simulink model "Integration_1_1"  (R2024b)
settings: Solver=VariableStepAuto  StartTime=0.0  StopTime=4  RelTol=1e-3
undefined symbols (not defined in the file): Ion, Lithium, Ts_Control
libraries: ee_lib x30, nesl_utility x24, spsSeriesRLCBranchLib x22, simulink x21, slpidlib x18, spsParallelRLCBranchLib x18, spsCurrentVoltageSimscapeInterfaceLib x18, powerlib_extras x18, spsThreePhaseVIMeasurementLib x7, spsGroundLib x7, spsThreePhaseSeriesRLCBranchLib x7, spsBoostConverterLib x6
(part 1 of 5)
settings Model: Creator=DELL  LastModifiedBy=mitphanase
settings DataIOCC: ReturnWorkspaceOutputs=off

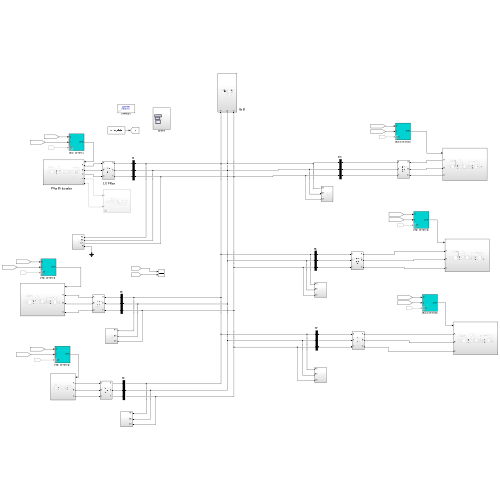
[thumbnail: Simulink's stored preview of the top-level diagram]
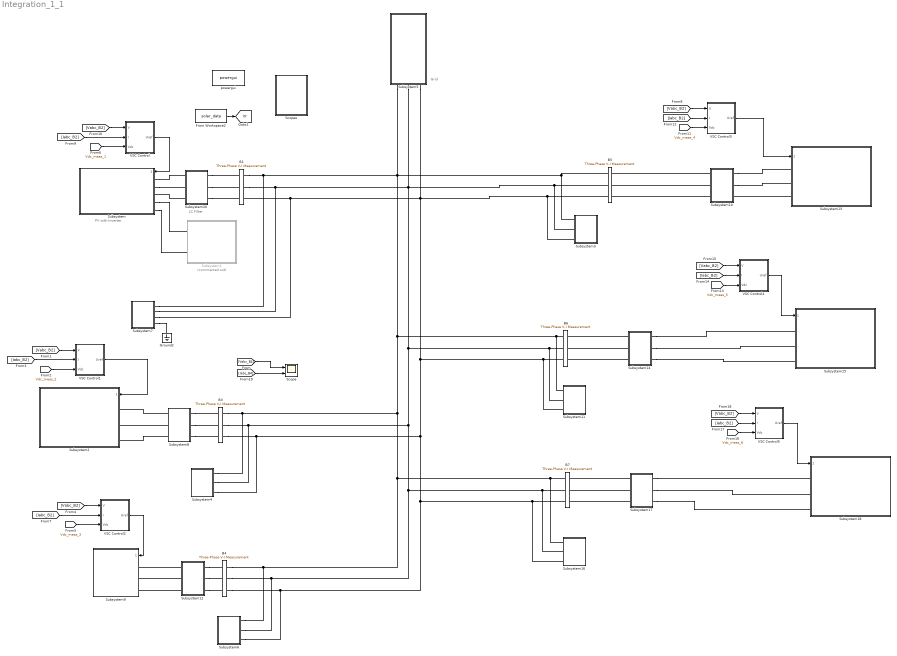
== system Integration_1_1 ==
  note: LC Filter
  note: Grid
  note: PV with Inverter
  B1 : spsThreePhaseVIMeasurementLib/Three-Phase V-I Measurement  VoltageMeasurement=phase-to-ground  SetLabelV=on  LabelV=Vabc_B1  Vpu=off  VpuLL=off  CurrentMeasurement=yes  SetLabelI=on  LabelI=Iabc_B1  Ipu=off  Pbase=100e6  Vbase=1000  OutputType=Magnitude  PhasorSimulation=off  PSBequivalent=0
  B3 : spsThreePhaseVIMeasurementLib/Three-Phase V-I Measurement  VoltageMeasurement=phase-to-ground  SetLabelV=on  LabelV=Vabc_B3  Vpu=off  VpuLL=off  CurrentMeasurement=yes  SetLabelI=on  LabelI=Iabc_B3  Ipu=off  Pbase=100e6  Vbase=1000  OutputType=Magnitude  PhasorSimulation=off  PSBequivalent=0
  B4 : spsThreePhaseVIMeasurementLib/Three-Phase V-I Measurement  VoltageMeasurement=phase-to-phase  SetLabelV=on  LabelV=Vabc_B4  Vpu=off  VpuLL=off  CurrentMeasurement=yes  SetLabelI=on  LabelI=Iabc_B4  Ipu=off  Pbase=100e6  Vbase=1000  OutputType=Magnitude  PhasorSimulation=off  PSBequivalent=0
  B5 : spsThreePhaseVIMeasurementLib/Three-Phase V-I Measurement  VoltageMeasurement=phase-to-phase  SetLabelV=on  LabelV=Vabc_B5  Vpu=off  VpuLL=off  CurrentMeasurement=yes  SetLabelI=on  LabelI=Iabc_B5  Ipu=off  Pbase=100e6  Vbase=1000  OutputType=Magnitude  PhasorSimulation=off  PSBequivalent=0
  B6 : spsThreePhaseVIMeasurementLib/Three-Phase V-I Measurement  VoltageMeasurement=phase-to-phase  SetLabelV=on  LabelV=Vabc_B6  Vpu=off  VpuLL=off  CurrentMeasurement=yes  SetLabelI=on  LabelI=Iabc_B6  Ipu=off  Pbase=100e6  Vbase=1000  OutputType=Magnitude  PhasorSimulation=off  PSBequivalent=0
  B7 : spsThreePhaseVIMeasurementLib/Three-Phase V-I Measurement  VoltageMeasurement=phase-to-phase  SetLabelV=on  LabelV=Vabc_B7  Vpu=off  VpuLL=off  CurrentMeasurement=yes  SetLabelI=on  LabelI=Iabc_B7  Ipu=off  Pbase=100e6  Vbase=1000  OutputType=Magnitude  PhasorSimulation=off  PSBequivalent=0
  From Workspace2 : FromWorkspace  VariableName=solar_data  OutDataTypeStr=double  SampleTime=0.01
  Ground2 : spsGroundLib/Ground  LConnTagsString=a
  Scope : Scope  NumInputPorts=2
  Scopes : Subsystem
  Subsystem : Subsystem
  Subsystem1 : Subsystem  Commented=on
  Subsystem10 : Subsystem
  Subsystem11 : Subsystem
  Subsystem12 : Subsystem
  Subsystem13 : Subsystem
  Subsystem14 : Subsystem
  Subsystem15 : Subsystem
  Subsystem16 : Subsystem
  Subsystem17 : Subsystem
  Subsystem18 : Subsystem
  Subsystem2 : Subsystem
  Subsystem20 : Subsystem
  Subsystem3 : Subsystem
  Subsystem4 : Subsystem
  Subsystem5 : Subsystem
  Subsystem6 : Subsystem
  Subsystem7 : Subsystem
  Subsystem8 : Subsystem
  Subsystem9 : Subsystem
  VSC Control : Subsystem  mask(VSC Main Controller){nom=[ 17e3  50 ], Vnom=[ 400 400 ], Vnom_dc=700, RLxfo=[0  0 ], RLchoke=[0  0  ], K_VDCreg=[18  600], K_Ireg=[0.2 20], Ts=Ts_Control}
      mask prompts: nom "Nominal power and frequency [ Pnom(VA)  Fnom(Hz) ]:"; Vnom "Nominal primary and secondary voltages (Vrms LL) [ Vnom_prim   Vnom_sec ]:"; Vnom_dc "Nominal DC bus voltage (V):"; RLxfo "Total transformer leakage impedance (pu/Pnom) [ Rxfo  Lxf ]"; RLchoke "Choke impedance [ R(ohm) L(H) ]"; K_VDCreg "VDC regultator gains [ Kp  Ki ]:"; K_Ireg "Current regulator gains [ Kp  Ki ]:"; Ts "Sample time"
      mask init:
      | Pnom=nom(1);
      | Fnom=nom(2);
      | Vnom_prim=Vnom(1);
      | Vnom_sec=Vnom(2);
      | Zbase=Vnom_sec^2/Pnom;
      | Rtot_pu=RLxfo(1) + RLchoke(1)/Zbase;
      | Ltot_pu=RLxfo(2) + RLchoke(2)/(Zbase/(2*pi*Fnom));
      | Kp_VDCreg=K_VDCreg(1);
      | Ki_VDCreg=K_VDCreg(2);
      | Kp_Ireg=K_Ireg(1);
      | Ki_Ireg=K_Ireg(2);
      | Vdc_ref=Vnom_dc;
  VSC Control1 : Subsystem  mask(VSC Main Controller){nom=[11e3  50 ], Vnom=[ 400 400 ], Vnom_dc=600, RLxfo=[0  0 ], RLchoke=[0  0  ], K_VDCreg=[18  600], K_Ireg=[0.2 20], Ts=Ts_Control}
      mask prompts: nom "Nominal power and frequency [ Pnom(VA)  Fnom(Hz) ]:"; Vnom "Nominal primary and secondary voltages (Vrms LL) [ Vnom_prim   Vnom_sec ]:"; Vnom_dc "Nominal DC bus voltage (V):"; RLxfo "Total transformer leakage impedance (pu/Pnom) [ Rxfo  Lxf ]"; RLchoke "Choke impedance [ R(ohm) L(H) ]"; K_VDCreg "VDC regultator gains [ Kp  Ki ]:"; K_Ireg "Current regulator gains [ Kp  Ki ]:"; Ts "Sample time"
      mask init: same as Integration_1_1/VSC Control
  VSC Control2 : Subsystem  mask(VSC Main Controller){nom=[ 7e3  50 ], Vnom=[ 400 400 ], Vnom_dc=600, RLxfo=[0  0 ], RLchoke=[0  0  ], K_VDCreg=[18  600], K_Ireg=[0.2 20], Ts=Ts_Control}
      mask prompts: nom "Nominal power and frequency [ Pnom(VA)  Fnom(Hz) ]:"; Vnom "Nominal primary and secondary voltages (Vrms LL) [ Vnom_prim   Vnom_sec ]:"; Vnom_dc "Nominal DC bus voltage (V):"; RLxfo "Total transformer leakage impedance (pu/Pnom) [ Rxfo  Lxf ]"; RLchoke "Choke impedance [ R(ohm) L(H) ]"; K_VDCreg "VDC regultator gains [ Kp  Ki ]:"; K_Ireg "Current regulator gains [ Kp  Ki ]:"; Ts "Sample time"
      mask init: same as Integration_1_1/VSC Control
  VSC Control3 : Subsystem  mask(VSC Main Controller){nom=[ 12.5e3  50 ], Vnom=[ 400 400 ], Vnom_dc=600, RLxfo=[0  0 ], RLchoke=[0  0  ], K_VDCreg=[12  600], K_Ireg=[0.2 20], Ts=Ts_Control}
      mask prompts: nom "Nominal power and frequency [ Pnom(VA)  Fnom(Hz) ]:"; Vnom "Nominal primary and secondary voltages (Vrms LL) [ Vnom_prim   Vnom_sec ]:"; Vnom_dc "Nominal DC bus voltage (V):"; RLxfo "Total transformer leakage impedance (pu/Pnom) [ Rxfo  Lxf ]"; RLchoke "Choke impedance [ R(ohm) L(H) ]"; K_VDCreg "VDC regultator gains [ Kp  Ki ]:"; K_Ireg "Current regulator gains [ Kp  Ki ]:"; Ts "Sample time"
      mask init: same as Integration_1_1/VSC Control
  VSC Control4 : Subsystem  mask(VSC Main Controller){nom=[ 8.5e3  50 ], Vnom=[ 400 400 ], Vnom_dc=600, RLxfo=[0  0 ], RLchoke=[0  0  ], K_VDCreg=[18  600], K_Ireg=[0.2 20], Ts=Ts_Control}
      mask prompts: nom "Nominal power and frequency [ Pnom(VA)  Fnom(Hz) ]:"; Vnom "Nominal primary and secondary voltages (Vrms LL) [ Vnom_prim   Vnom_sec ]:"; Vnom_dc "Nominal DC bus voltage (V):"; RLxfo "Total transformer leakage impedance (pu/Pnom) [ Rxfo  Lxf ]"; RLchoke "Choke impedance [ R(ohm) L(H) ]"; K_VDCreg "VDC regultator gains [ Kp  Ki ]:"; K_Ireg "Current regulator gains [ Kp  Ki ]:"; Ts "Sample time"
      mask init: same as Integration_1_1/VSC Control
  VSC Control5 : Subsystem  mask(VSC Main Controller){nom=[ 10e3  50 ], Vnom=[ 400 400 ], Vnom_dc=600, RLxfo=[0  0 ], RLchoke=[0  0  ], K_VDCreg=[18  600], K_Ireg=[0.2 20], Ts=Ts_Control}
      mask prompts: nom "Nominal power and frequency [ Pnom(VA)  Fnom(Hz) ]:"; Vnom "Nominal primary and secondary voltages (Vrms LL) [ Vnom_prim   Vnom_sec ]:"; Vnom_dc "Nominal DC bus voltage (V):"; RLxfo "Total transformer leakage impedance (pu/Pnom) [ Rxfo  Lxf ]"; RLchoke "Choke impedance [ R(ohm) L(H) ]"; K_VDCreg "VDC regultator gains [ Kp  Ki ]:"; K_Ireg "Current regulator gains [ Kp  Ki ]:"; Ts "Sample time"
      mask init: same as Integration_1_1/VSC Control
  powergui : sps_lib/powergui  Priority=1  SimulationMode=Discrete  SampleTime=1e-4  frequency=60  Iterations=50  frequencyindice=0  Pbase=100e6  ErrMax=1e-4  UnitsV=kV  UnitsW=MW  buscounter=0  FunctionMessages=off  echomessages=off  EnableUseOfTLC=off  CurrentSourceSwitches=off  DisableSnubberDevices=off  DisableRonSwitches=off  DisableVfSwitches=off  DisplayEquations=off  AutomaticDiscreteSolvers=off  SolverType=Tustin/Backward Euler (TBE)  Interpol=off  ExternalGateDelay=off  methode=off  Ts=100  x0status=blocks  SPID=on  SwTol=0  HookPort=off  NonlinearTolerance=1e-4  nMaxIteration=100  ContinueOnMaxIteration=off  RestoreLinks=warning  ResistiveCurrentMeasurement=off  Frange=[0:2:500]  Ylog=off  Xlog=on  ShowGrid=off  save=off  variable=ZData  structure=0  ZoomFFT=off  StartTime=0.0  cycles=1  DisplayStyle=1  fundamental=60  FreqAxis=off  MaxFrequency=1000  frequencyindicesteady=1  RmsSteady=1  display=off
  tag scope: irr=global
  wires:
  [Vdc_meas_1] -> VSC Control/3(Vdc)
  [Vabc_B2] -> VSC Control/1(V)
  [Iabc_B2] -> VSC Control/2(I)
  VSC Control/1(Uref) -> Subsystem/1("  ")
  From Workspace2/1 -> [irr]
  [Vabc_B2] -> VSC Control2/1(V)
  [Vdc_meas_3] -> VSC Control2/3(Vdc)
  [Iabc_B2] -> VSC Control2/2(I)
  VSC Control2/1(Uref) -> Subsystem9/1("  ")
  VSC Control3/1(Uref) -> Subsystem13/1("  ")
  [Vabc_B2] -> VSC Control3/1(V)
  [Iabc_B2] -> VSC Control3/2(I)
  [Vdc_meas_4] -> VSC Control3/3(Vdc)
  [Vdc_meas_5] -> VSC Control4/3(Vdc)
  [Iabc_B2] -> VSC Control4/2(I)
  [Vabc_B2] -> VSC Control4/1(V)
  VSC Control4/1(Uref) -> Subsystem15/1("  ")
  VSC Control5/1(Uref) -> Subsystem18/1("  ")
  [Vabc_B2] -> VSC Control5/1(V)
  [Iabc_B2] -> VSC Control5/2(I)
  [Vdc_meas_6] -> VSC Control5/3(Vdc)
  VSC Control1/1(Uref) -> Subsystem2/1("  ")
  [Iabc_B2] -> VSC Control1/2(I)
  [Vdc_meas_2] -> VSC Control1/3(Vdc)
  [Vabc_B2] -> VSC Control1/1(V)
  [Vabc_B4] -> Scope/1
  [Iabc_B4] -> Scope/2
  connections:
  Subsystem12/RConn1 -- B4/LConn1
  Subsystem12/LConn2 -- Subsystem9/LConn2
  Subsystem12/RConn3 -- B4/LConn3
  Subsystem12/LConn3 -- Subsystem9/LConn3
  Subsystem12/LConn1 -- Subsystem9/LConn1
  Subsystem12/RConn2 -- B4/LConn2
  Subsystem14/LConn2 -- Subsystem15/LConn2
  Subsystem14/RConn3 -- B6/LConn3
  Subsystem14/LConn1 -- Subsystem15/LConn1
  Subsystem14/LConn3 -- Subsystem15/LConn3
  Subsystem14/RConn1 -- B6/LConn1
  Subsystem14/RConn2 -- B6/LConn2
  Subsystem17/LConn2 -- Subsystem18/LConn2
  Subsystem17/RConn3 -- B7/LConn3
  Subsystem17/LConn1 -- Subsystem18/LConn1
  Subsystem17/LConn3 -- Subsystem18/LConn3
  Subsystem17/RConn1 -- B7/LConn1
  Subsystem17/RConn2 -- B7/LConn2
  Subsystem10/RConn1 -- B5/LConn1
  Subsystem10/RConn2 -- B5/LConn2
  Subsystem10/RConn3 -- B5/LConn3
  Subsystem10/LConn2 -- Subsystem13/LConn2
  Subsystem10/LConn1 -- Subsystem13/LConn1
  Subsystem13/LConn3 -- Subsystem10/LConn3
  Subsystem5/LConn2 -- Subsystem7/LConn2 -- B1/RConn2 -- Subsystem4/LConn2 -- B3/RConn2 -- Subsystem6/LConn2 -- B4/RConn2 -- Subsystem16/LConn2 -- B7/RConn2 -- Subsystem11/LConn2 -- B6/RConn2 -- Subsystem3/LConn2 -- B5/RConn2
  Subsystem20/LConn1 -- Subsystem/LConn1
  Subsystem/LConn2 -- Subsystem20/LConn2
  Subsystem20/LConn3 -- Subsystem/LConn3
  Subsystem20/RConn1 -- B1/LConn1
  Subsystem20/RConn2 -- B1/LConn2
  Subsystem20/RConn3 -- B1/LConn3
  Subsystem7/LConn4 -- Ground2/LConn1
  Subsystem/LConn4 -- Subsystem1/LConn1
  Subsystem/LConn5 -- Subsystem1/LConn2
  Subsystem8/LConn2 -- Subsystem2/LConn2
  Subsystem8/LConn3 -- Subsystem2/LConn3
  Subsystem8/LConn1 -- Subsystem2/LConn1
  Subsystem8/RConn1 -- B3/LConn1
  Subsystem8/RConn2 -- B3/LConn2
  Subsystem8/RConn3 -- B3/LConn3
  Subsystem5/LConn1 -- B5/RConn1 -- Subsystem3/LConn1 -- Subsystem7/LConn1 -- B1/RConn1 -- Subsystem4/LConn1 -- B3/RConn1 -- Subsystem6/LConn1 -- B4/RConn1 -- Subsystem16/LConn1 -- B7/RConn1 -- Subsystem11/LConn1 -- B6/RConn1
  Subsystem5/LConn3 -- Subsystem7/LConn3 -- B1/RConn3 -- Subsystem4/LConn3 -- B3/RConn3 -- Subsystem6/LConn3 -- B4/RConn3 -- Subsystem16/LConn3 -- B7/RConn3 -- Subsystem11/LConn3 -- B6/RConn3 -- Subsystem3/LConn3 -- B5/RConn3

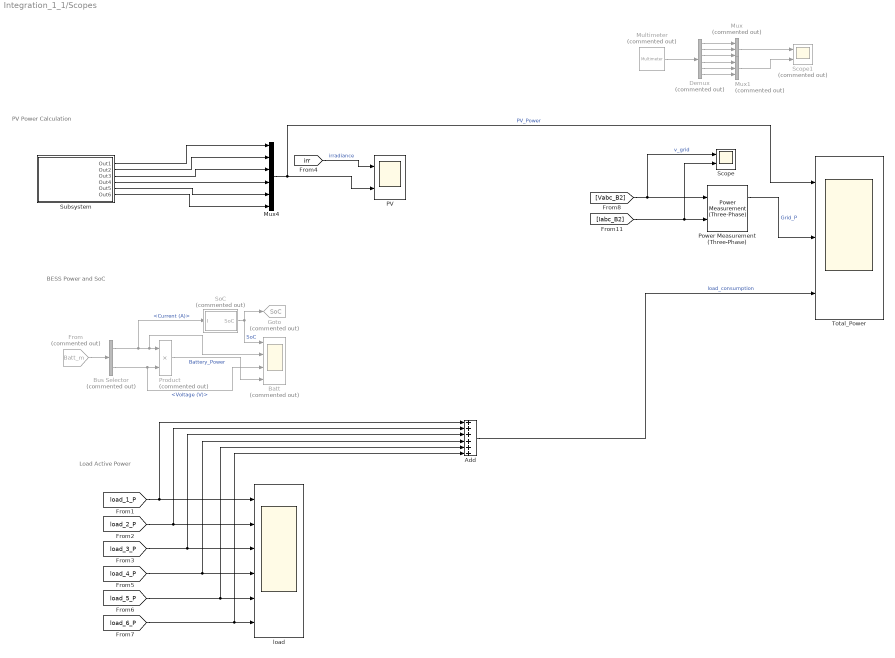
== system Integration_1_1/Scopes ==
  note: Load Active Power
  note: BESS Power and SoC
  note: PV Power Calculation
  Add : Sum  Inputs=++++++
  Batt : Scope  Commented=on  NumInputPorts=4
  Bus Selector : BusSelector  Commented=on  OutputSignals=Current (A),Voltage (V)
  Demux : Demux  Commented=on  Outputs=6
  From : From  Commented=on  GotoTag=Batt_m
  Goto : Goto  Commented=on  GotoTag=SoC  TagVisibility=global
  Multimeter : spsMultimeterLib/Multimeter  Commented=on  L=2  sel=1  yselected={}  Gain=0  OutputType=Complex  PlotAtSimulationStop=off  PhasorSimulation=off
  Mux : Mux  Commented=on  Inputs=3
  Mux1 : Mux  Commented=on  Inputs=3
  Mux4 : Mux  Inputs=6
  PV : Scope  NumInputPorts=2
  Power Measurement (Three-Phase) : eePowerMeasurement/Power Measurement (Three-Phase)  LabelModeActiveChoice=Discrete  F=50  K=[1]  Seq=Positive  Ts=Ts_Control
  Product : Product  Commented=on
  Scope : Scope  NumInputPorts=2
  Scope1 : Scope  Commented=on  NumInputPorts=2
  SoC : Subsystem  Commented=on
  Subsystem : Subsystem
  Total_Power : Scope  NumInputPorts=3
  load : Scope  NumInputPorts=6
  wires:
  [irr] -> PV/1  "irradiance"
  SoC/1(SoC) -> Goto/1, Batt/1  "SoC"
  Subsystem/1(Out1) -> Mux4/1
  Subsystem/2(Out2) -> Mux4/2
  Subsystem/3(Out3) -> Mux4/3
  Subsystem/4(Out4) -> Mux4/4
  Subsystem/5(Out5) -> Mux4/5
  Subsystem/6(Out6) -> Mux4/6
  Mux4/1 -> PV/2, Total_Power/1  "PV_Power"
  From/1 -> Bus Selector/1
  Bus Selector/1 -> SoC/1(I), Batt/2, Product/1  "<Current (A)>"
  Bus Selector/2 -> Batt/3, Product/2  "<Voltage (V)>"
  Product/1 -> Batt/4  "Battery_Power"
  [load_1_P] -> Add/1, load/1
  [load_4_P] -> Add/4, load/4
  [load_3_P] -> Add/3, load/3
  [load_2_P] -> Add/2, load/2
  [load_5_P] -> Add/5, load/5
  [load_6_P] -> Add/6, load/6
  [Vabc_B2] -> Scope/1, Power Measurement (Three-Phase)/1  "v_grid"
  [Iabc_B2] -> Scope/2, Power Measurement (Three-Phase)/2
  Power Measurement (Three-Phase)/1 -> Total_Power/2  "Grid_P"
  Multimeter/1 -> Demux/1
  Demux/1 -> Mux/1
  Demux/2 -> Mux/2
  Mux/1 -> Scope1/1
  Demux/3 -> Mux/3
  Demux/4 -> Mux1/1
  Demux/5 -> Mux1/2
  Demux/6 -> Mux1/3
  Mux1/1 -> Scope1/2
  Add/1 -> Total_Power/3  "load_consumption"

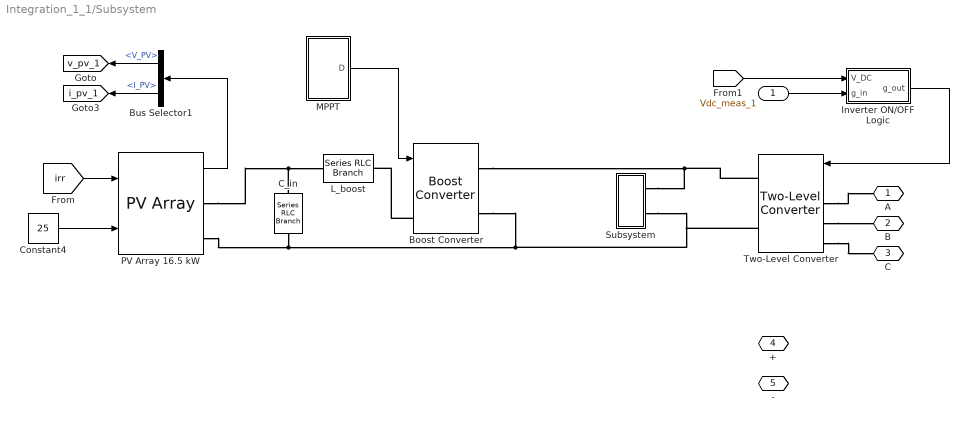
== system Integration_1_1/Subsystem ==
  "  " : Inport
  Boost Converter : spsBoostConverterLib/Boost Converter  ModelType=Average model (D-controlled)  Ron=1e-3  Rs=1e6  Cs=inf  Vforward=[0,0]  Ron_Diode=1e-3  Rs_Diode=1e6  Cs_Diode=inf  Vf_Diode=1e-3  Rs_CurrentSource=inf  Ron_ACsource=1e-3
      settings: LibrarySourceBlock=sps_lib/Power Electronics/Boost Converter
  Bus Selector1 : BusSelector  OutputSignals=V_PV,I_PV
  C_in : spsSeriesRLCBranchLib/Series RLC Branch  LConnTagsString=__new0  RConnTagsString=__new0  BranchType=C  Resistance=1e-5  Inductance=1e-3  SetiL0=off  InitialCurrent=0  Capacitance=850e-6  Setx0=off  InitialVoltage=426.5  Measurements=Branch voltage and current
  Constant4 : Constant  Value=25
  Inverter ON/OFF Logic : Subsystem
  L_boost : spsSeriesRLCBranchLib/Series RLC Branch  LConnTagsString=__new0  RConnTagsString=__new0  BranchType=L  Resistance=1e-3  Inductance=70e-3  SetiL0=off  InitialCurrent=0  Capacitance=100e-6  Setx0=off  InitialVoltage=230  Measurements=None
  MPPT : Subsystem
  PV Array 16.5 kW : spsPVArrayLib/PV Array  Npar=8  Nser=5  PlotType=array @ 1000 W/m2 & specified temperatures  S_vec="[ 1000  500  100 ]"  Temp_C_vec="[ 45 25  ]"  ModuleName=SunPower SPR-415E-WHT-D  PlotWhenSelected=off  Pm=414.801  Ncell=128  Voc=85.3  Isc=6.09  Vm=72.9  Im=5.69  beta_Voc_pc=-0.229  alpha_Isc_pc=0.030706  beta_Voc=-0.19534  alpha_Isc=0.00187  IL=6.0978  I0=7.1698e-13  nI=0.87223  Rsh=419.7781  Rs=0.53711  RobustModel=off  RobustCellTemperature=313.3991  BAL=on  Tc=1e-6  Tfilter=5e-5
  Subsystem : Subsystem
  Two-Level Converter : spsTwoLevelConverterLib/Two-Level Converter  ModelType=Average model (No rectifier mode)  Ron=1e-3  Rs=1e6  Cs=inf  Vforward=[0,0]  Ron_Diode=1e-3  Rs_Diode=1e6  Cs_Diode=inf  Vf_Diode=1e-3  Rs_CurrentSource=inf  Ron_ACsource=1e-3
      settings: LibrarySourceBlock=sps_lib/Power Electronics/Two-Level Converter
  A : PMIOPort  Side=Left
  B : PMIOPort  Port=2  Side=Left
  C : PMIOPort  Port=3  Side=Left
  + : PMIOPort  Port=4  Side=Left
  - : PMIOPort  Port=5  Side=Left
  tag scope: i_pv_1=global, v_pv_1=global
  wires:
  Bus Selector1/1 -> [v_pv_1]  "<V_PV>"
  Bus Selector1/2 -> [i_pv_1]  "<I_PV>"
  PV Array 16.5 kW/1 -> Bus Selector1/1
  [irr] -> PV Array 16.5 kW/1
  MPPT/1(D) -> Boost Converter/1
  "  "/1 -> Inverter ON/OFF Logic/2(g_in)
  Inverter ON/OFF Logic/1(g_out) -> Two-Level Converter/1
  Constant4/1 -> PV Array 16.5 kW/2
  [Vdc_meas_1] -> Inverter ON/OFF Logic/1(V_DC)
  connections:
  Two-Level Converter/LConn1 -- A/RConn1
  PV Array 16.5 kW/RConn2 -- C_in/RConn1 -- Two-Level Converter/RConn2 -- Subsystem/RConn2 -- Boost Converter/RConn2
  PV Array 16.5 kW/RConn1 -- C_in/LConn1 -- L_boost/LConn1
  Boost Converter/RConn1 -- Two-Level Converter/RConn1 -- Subsystem/RConn1
  Two-Level Converter/LConn3 -- C/RConn1
  Two-Level Converter/LConn2 -- B/RConn1
  Boost Converter/LConn1 -- L_boost/RConn1

== system Integration_1_1/Subsystem1 ==
  BATT chg-dshg logic1 : Subsystem
  Battery : spsBatteryLib/Battery  BatType=Lithium-Ion  NomV=48  NomQ=100  SOC=0  Batt_Tr=46.3e-3  PresetModel=on  MaxQ=100  MinV=36  FullV=55.8714  Dis_rate=43.4783  R=0.0048  Normal_OP=90.4348  expZone="[51.8585      4.91304]"
  Current Measurement : spsCurrentMeasurementLib/Current Measurement  PhasorSimulation=off  OutputType=Complex  PSBequivalent=0
  L_B : spsSeriesRLCBranchLib/Series RLC Branch  LConnTagsString=__new0  RConnTagsString=__new0  BranchType=L  Resistance=1e-3  Inductance=5e-3  SetiL0=off  InitialCurrent=0  Capacitance=100e-6  Setx0=off  InitialVoltage=230  Measurements=None
  Two-Quadrant DC/DC Converter : spsTwoQuadrantDCDCConverterLib/Two-Quadrant DC//DC Converter  ModelType=Average model (D-controlled)  Ron=1e-3  Rs=1e6  Cs=inf  Vforward=[0,0]  Ron_Diode=1e-3  Rs_Diode=1e6  Cs_Diode=inf  Vf_Diode=1e-3  Rs_CurrentSource=inf  Ron_ACsource=1e-3
  + : PMIOPort  Side=Left
  - : PMIOPort  Port=2  Side=Left
  tag scope: Batt_m=global
  wires:
  BATT chg-dshg logic1/1(D) -> Two-Quadrant DC/DC Converter/1
  Battery/1 -> [Batt_m]
  Current Measurement/1 -> BATT chg-dshg logic1/1(I_B)
  connections:
  Two-Quadrant DC/DC Converter/RConn1 -- +/RConn1
  Battery/LConn2 -- Two-Quadrant DC/DC Converter/RConn2 -- -/RConn1
  L_B/RConn1 -- Two-Quadrant DC/DC Converter/LConn1
  Current Measurement/RConn1 -- Battery/LConn1
  Current Measurement/LConn1 -- L_B/LConn1

== system Integration_1_1/Subsystem10 ==
  Parallel RLC Branch : spsParallelRLCBranchLib/Parallel RLC Branch  LConnTagsString=a  RConnTagsString=__new0  BranchType=RC  Resistance=68  Inductance=1e-3  SetiL0=off  InitialCurrent=0  Capacitance=0.81e-6  Setx0=off  InitialVoltage=0  Measurements=None
  Parallel RLC Branch1 : spsParallelRLCBranchLib/Parallel RLC Branch  LConnTagsString=a  RConnTagsString=__new0  BranchType=RC  Resistance=68  Inductance=1e-3  SetiL0=off  InitialCurrent=0  Capacitance=0.81e-6  Setx0=off  InitialVoltage=0  Measurements=None
  Parallel RLC Branch2 : spsParallelRLCBranchLib/Parallel RLC Branch  LConnTagsString=a  RConnTagsString=__new0  BranchType=RC  Resistance=68  Inductance=1e-3  SetiL0=off  InitialCurrent=0  Capacitance=0.81e-6  Setx0=off  InitialVoltage=0  Measurements=None
  Three-Phase Series RLC Branch1 : spsThreePhaseSeriesRLCBranchLib/Three-Phase Series RLC Branch  LConnTagsString=A|B|C  RConnTagsString=A|B|C  BranchType=L  Resistance=1  Inductance=3*3.71e-3  Capacitance=1e-6  Measurements=None
  A : PMIOPort  Side=Left
  B : PMIOPort  Port=2  Side=Left
  C : PMIOPort  Port=3  Side=Left
  a : PMIOPort  Port=4  Side=Right
  b : PMIOPort  Port=5  Side=Right
  c : PMIOPort  Port=6  Side=Right
  connections:
  c/RConn1 -- Three-Phase Series RLC Branch1/RConn3 -- Parallel RLC Branch2/LConn1 -- Parallel RLC Branch1/RConn1
  Three-Phase Series RLC Branch1/LConn3 -- C/RConn1
  Three-Phase Series RLC Branch1/LConn2 -- B/RConn1
  Three-Phase Series RLC Branch1/LConn1 -- A/RConn1
  a/RConn1 -- Three-Phase Series RLC Branch1/RConn1 -- Parallel RLC Branch2/RConn1 -- Parallel RLC Branch/LConn1
  b/RConn1 -- Parallel RLC Branch1/LConn1 -- Parallel RLC Branch/RConn1 -- Three-Phase Series RLC Branch1/RConn2

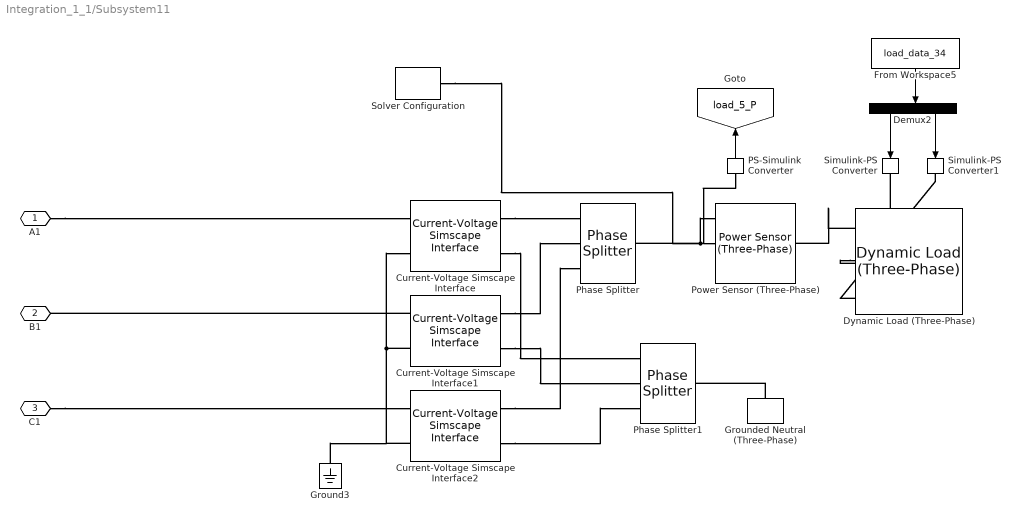
== system Integration_1_1/Subsystem11 ==
  Current-Voltage Simscape Interface : spsCurrentVoltageSimscapeInterfaceLib/Current-Voltage Simscape Interface  DFT=off  FMode=Low pass filter (continuous)  T=1e-4  Ts=50e-6  i0=0  v0=0  Sd=Specialized Power Systems side  Measurements=off
  Current-Voltage Simscape Interface1 : spsCurrentVoltageSimscapeInterfaceLib/Current-Voltage Simscape Interface  DFT=off  FMode=Low pass filter (continuous)  T=1e-4  Ts=50e-6  i0=0  v0=0  Sd=Specialized Power Systems side  Measurements=off
  Current-Voltage Simscape Interface2 : spsCurrentVoltageSimscapeInterfaceLib/Current-Voltage Simscape Interface  DFT=off  FMode=Low pass filter (continuous)  T=1e-4  Ts=50e-6  i0=0  v0=0  Sd=Specialized Power Systems side  Measurements=off
  Demux2 : Demux  Outputs=2
  Dynamic Load (Three-Phase) : ee_lib/Passive/Dynamic Load (Three-Phase)  port_option=ee.enum.threePhasePort.composite  FRated=50 Hz  Vline_rms_min=400 V  tau=0.01 s  Vline_rms_ini=400 V  Vang_ini=0 deg  gmin=0 S  fault_action=simscape.enum.assert.action.none  t_fault=1 s
      settings: InternalSimscapePortConfiguration="{\"Bottom\":[],\"Left\":[{\"id\":\"N\",\"label\":\"~\",\"type\":\"foundation.electrical.three_phase\"}],\"Right\":[],\"Top\":[{\"id\":\"P\",\"label\":\"P\",\"type\":\"input\"},{\"id\":\"Q\",\"label\":\"Q\",\"type\":\"input\"}]}"
  From Workspace5 : FromWorkspace  VariableName=load_data_34  SampleTime=0.01
  Ground3 : spsGroundLib/Ground  LConnTagsString=a
  Grounded Neutral (Three-Phase) : ee_lib/Connectors & References/Grounded Neutral (Three-Phase)
  PS-Simulink Converter : nesl_utility/PS-Simulink Converter  PhysicalDomain=network_engine_domain  SubClassName=ps_output  LeftPortType=input  RightPortType=output  PseudoPeriodic=off  Frequencies=[]  VectorFormat=inherit  Unit=inherit  AffineConversion=off
  Phase Splitter : ee_lib/Connectors & References/Phase Splitter
  Phase Splitter1 : ee_lib/Connectors & References/Phase Splitter
  Power Sensor (Three-Phase) : ee_lib/Sensors & Transducers/Power Sensor (Three-Phase)  load_type=ee.enum.passive.type_balanced.unbalanced  f0=50 Hz  config=ee.enum.with_neutral.no  rho=1
      settings: InternalSimscapePortConfiguration="{\"Bottom\":[],\"Left\":[{\"id\":\"N1\",\"label\":\"~1\",\"type\":\"foundation.electrical.three_phase\"}],\"Right\":[{\"id\":\"N2\",\"label\":\"~2\",\"type\":\"foundation.electrical.three_phase\"}],\"Top\":[{\"id\":\"Pm\",\"label\":\"P\",\"type\":\"output\"},{\"id\":\"Qm\",\"label\":\"Q\",\"type\":\"output\"}]}"
  Simulink-PS Converter : nesl_utility/Simulink-PS Converter  PhysicalDomain=network_engine_domain  SubClassName=ps_input  LeftPortType=input  RightPortType=output  PseudoPeriodic=off  Frequencies=[]  NoiseDistribution=none  NoiseParameters=[]  Unit=1  AffineConversion=off  FilteringAndDerivatives=provide  SimscapeFilterOrder=1  InputFilterTimeConstant=0.001  UdotUserProvided=0
  Simulink-PS Converter1 : nesl_utility/Simulink-PS Converter  PhysicalDomain=network_engine_domain  SubClassName=ps_input  LeftPortType=input  RightPortType=output  PseudoPeriodic=off  Frequencies=[]  NoiseDistribution=none  NoiseParameters=[]  Unit=1  AffineConversion=off  FilteringAndDerivatives=provide  SimscapeFilterOrder=1  InputFilterTimeConstant=0.001  UdotUserProvided=0
  Solver Configuration : nesl_utility/Solver Configuration  PhysicalDomain=network_engine_domain  SubClassName=solver  LeftPortType=input  RightPortType=generic  Tones=[]  Harmonics=[]  SimulateNoise=off  Profile=off  UseLocalSampling=off  EnableSwitchedLinearOptims=on  FrequencyDomain=off  UseCCode=off  RelTol=0.001  AbsTol=0.001  MinStep=1e-09  ToWorkspace=off  RevertToSquareIcSolve=off  NumHomotopyIterations=100  PhasorMode=off  PhasorModeNumHarmonics=1  ConsistencySolver=NEWTON_XTOL_AFTER_FTOL  IndexReductionMethod=DerivativeReplacement  DoDC=on  ResidualTolerance=1e-09  ConsistencyTolSource=GLOBAL  ConsistencyAbsTol=0.001  ConsistencyRelTol=0.001  ConsistencyTolFactor=0.001  UseLocalSolver=off  LocalSolverChoice=NE_BACKWARD_EULER_ADVANCER  ResolveIndetEquations=on  FunctionEvalNumThread=1  LocalSolverSampleTime=0.0001  DoFixedCost=off  MaxNonlinIter=3  MaxModeIter=2  ComputeImpulses=off  ImpulseIterations=2  LinearAlgebra=Sparse  LinearAlgebraNumThread=0  EquationFormulation=NE_TIME_EF  DelaysMemoryBudget=1024  AutomaticFiltering=off  FilteringTimeConstant=0.001  PartitionStorageMethod=AS_NEEDED  PartitionMemoryBudget=1024  PartitionMethod=ROBUST  MultibodyUseLocalSolver=off  MultibodyLocalSolverChoice=ODE1  MultibodyLocalSolverSampleTime=0.001
  A1 : PMIOPort  Side=Left
  B1 : PMIOPort  Port=2  Side=Left
  C1 : PMIOPort  Port=3  Side=Left
  tag scope: load_5_P=global
  wires:
  From Workspace5/1 -> Demux2/1
  Demux2/2 -> Simulink-PS Converter1/1
  PS-Simulink Converter/1 -> [load_5_P]
  Demux2/1 -> Simulink-PS Converter/1
  connections:
  Power Sensor (Three-Phase)/LConn1 -- Solver Configuration/RConn1 -- Phase Splitter/LConn1
  Current-Voltage Simscape Interface1/RConn2 -- Phase Splitter1/RConn2
  Current-Voltage Simscape Interface2/RConn2 -- Phase Splitter1/RConn3
  Dynamic Load (Three-Phase)/LConn1 -- Power Sensor (Three-Phase)/RConn1
  Current-Voltage Simscape Interface1/RConn1 -- Phase Splitter/RConn2
  Current-Voltage Simscape Interface2/RConn1 -- Phase Splitter/RConn3
  Current-Voltage Simscape Interface/RConn1 -- Phase Splitter/RConn1
  Dynamic Load (Three-Phase)/LConn3 -- Simulink-PS Converter1/RConn1
  Grounded Neutral (Three-Phase)/LConn1 -- Phase Splitter1/LConn1
  Current-Voltage Simscape Interface/RConn2 -- Phase Splitter1/RConn1
  PS-Simulink Converter/LConn1 -- Power Sensor (Three-Phase)/LConn2
  Dynamic Load (Three-Phase)/LConn2 -- Simulink-PS Converter/RConn1
  A1/RConn1 -- Current-Voltage Simscape Interface/LConn1
  Current-Voltage Simscape Interface1/LConn1 -- B1/RConn1
  Current-Voltage Simscape Interface1/LConn2 -- Current-Voltage Simscape Interface2/LConn2 -- Ground3/LConn1 -- Current-Voltage Simscape Interface/LConn2
  C1/RConn1 -- Current-Voltage Simscape Interface2/LConn1

== system Integration_1_1/Subsystem12 ==
  Series RLC Branch1 : spsSeriesRLCBranchLib/Series RLC Branch  LConnTagsString=__new0  RConnTagsString=__new0  BranchType=RC  Resistance=10  Inductance=1e-3  SetiL0=off  InitialCurrent=0  Capacitance=0.41e-6  Setx0=off  InitialVoltage=0  Measurements=None
  Series RLC Branch2 : spsSeriesRLCBranchLib/Series RLC Branch  LConnTagsString=__new0  RConnTagsString=__new0  BranchType=RC  Resistance=10  Inductance=1e-3  SetiL0=off  InitialCurrent=0  Capacitance=0.41e-6  Setx0=off  InitialVoltage=0  Measurements=None
  Series RLC Branch3 : spsSeriesRLCBranchLib/Series RLC Branch  LConnTagsString=__new0  RConnTagsString=__new0  BranchType=RC  Resistance=10  Inductance=1e-3  SetiL0=off  InitialCurrent=0  Capacitance=0.41e-6  Setx0=off  InitialVoltage=0  Measurements=None
  Three-Phase Series RLC Branch1 : spsThreePhaseSeriesRLCBranchLib/Three-Phase Series RLC Branch  LConnTagsString=A|B|C  RConnTagsString=A|B|C  BranchType=L  Resistance=1  Inductance=7.423e-3  Capacitance=1e-6  Measurements=None
  A : PMIOPort  Side=Left
  B : PMIOPort  Port=2  Side=Left
  C : PMIOPort  Port=3  Side=Left
  a : PMIOPort  Port=4  Side=Right
  b : PMIOPort  Port=5  Side=Right
  c : PMIOPort  Port=6  Side=Right
  connections:
  Three-Phase Series RLC Branch1/RConn2 -- Series RLC Branch1/LConn1 -- Series RLC Branch3/RConn1 -- b/RConn1
  Series RLC Branch2/RConn1 -- Series RLC Branch3/LConn1 -- Three-Phase Series RLC Branch1/RConn1 -- a/RConn1
  Three-Phase Series RLC Branch1/LConn1 -- A/RConn1
  Three-Phase Series RLC Branch1/LConn2 -- B/RConn1
  Three-Phase Series RLC Branch1/LConn3 -- C/RConn1
  Series RLC Branch1/RConn1 -- Series RLC Branch2/LConn1 -- Three-Phase Series RLC Branch1/RConn3 -- c/RConn1

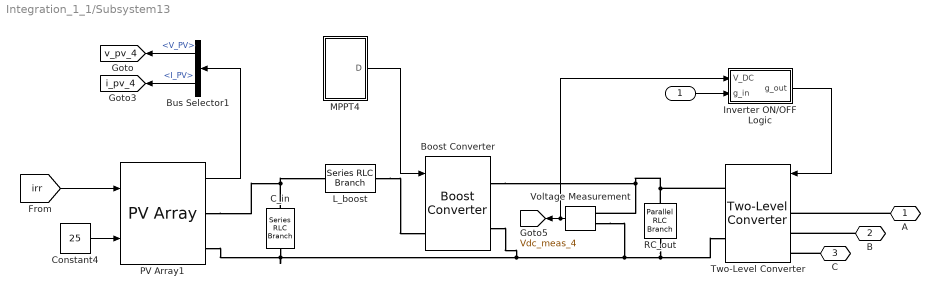
== system Integration_1_1/Subsystem13 ==
  "  " : Inport
  Boost Converter : spsBoostConverterLib/Boost Converter  ModelType=Average model (D-controlled)  Ron=1e-3  Rs=1e6  Cs=inf  Vforward=[0,0]  Ron_Diode=1e-3  Rs_Diode=1e6  Cs_Diode=inf  Vf_Diode=1e-3  Rs_CurrentSource=inf  Ron_ACsource=1e-3
      settings: LibrarySourceBlock=sps_lib/Power Electronics/Boost Converter
  Bus Selector1 : BusSelector  OutputSignals=V_PV,I_PV
  C_in : spsSeriesRLCBranchLib/Series RLC Branch  LConnTagsString=__new0  RConnTagsString=__new0  BranchType=C  Resistance=1e-5  Inductance=1e-3  SetiL0=off  InitialCurrent=0  Capacitance=628.37e-6  Setx0=off  InitialVoltage=426.5  Measurements=None
  Constant4 : Constant  Value=25
  Inverter ON/OFF Logic : Subsystem
  L_boost : spsSeriesRLCBranchLib/Series RLC Branch  LConnTagsString=__new0  RConnTagsString=__new0  BranchType=L  Resistance=1e-3  Inductance=78.31e-3  SetiL0=off  InitialCurrent=0  Capacitance=100e-6  Setx0=off  InitialVoltage=230  Measurements=None
  MPPT4 : Subsystem
  PV Array1 : spsPVArrayLib/PV Array  Npar=6  Nser=5  PlotType=array @ 1000 W/m2 & specified temperatures  S_vec="[ 1000  500  100 ]"  Temp_C_vec="[ 45 25  ]"  ModuleName=SunPower SPR-415E-WHT-D  PlotWhenSelected=off  Pm=414.801  Ncell=128  Voc=85.3  Isc=6.09  Vm=72.9  Im=5.69  beta_Voc_pc=-0.229  alpha_Isc_pc=0.030706  beta_Voc=-0.19534  alpha_Isc=0.00187  IL=6.0978  I0=7.1698e-13  nI=0.87223  Rsh=419.7781  Rs=0.53711  RobustModel=off  RobustCellTemperature=313.3991  BAL=on  Tc=1e-6  Tfilter=5e-5
  RC_out : spsParallelRLCBranchLib/Parallel RLC Branch  LConnTagsString=a  RConnTagsString=__new0  BranchType=RC  Resistance=50  Inductance=1e-3  SetiL0=off  InitialCurrent=0  Capacitance=478.065e-6  Setx0=off  InitialVoltage=700  Measurements=None
  Two-Level Converter : spsTwoLevelConverterLib/Two-Level Converter  ModelType=Average model (No rectifier mode)  Ron=1e-3  Rs=1e6  Cs=inf  Vforward=[0,0]  Ron_Diode=1e-3  Rs_Diode=1e6  Cs_Diode=inf  Vf_Diode=1e-3  Rs_CurrentSource=inf  Ron_ACsource=1e-3
  Voltage Measurement : spsVoltageMeasurementLib/Voltage Measurement  PhasorSimulation=off  OutputType=Complex  PSBequivalent=0
  A : PMIOPort  Side=Left
  B : PMIOPort  Port=2  Side=Left
  C : PMIOPort  Port=3  Side=Left
  tag scope: Vdc_meas_4=global, i_pv_4=global, v_pv_4=global
  wires:
  Voltage Measurement/1 -> Inverter ON/OFF Logic/1(V_DC), [Vdc_meas_4]
  Bus Selector1/1 -> [v_pv_4]  "<V_PV>"
  Constant4/1 -> PV Array1/2
  Bus Selector1/2 -> [i_pv_4]  "<I_PV>"
  PV Array1/1 -> Bus Selector1/1
  [irr] -> PV Array1/1
  MPPT4/1(D) -> Boost Converter/1
  Inverter ON/OFF Logic/1(g_out) -> Two-Level Converter/1
  "  "/1 -> Inverter ON/OFF Logic/2(g_in)
  connections:
  A/RConn1 -- Two-Level Converter/LConn1
  Two-Level Converter/RConn2 -- RC_out/RConn1 -- Boost Converter/RConn2 -- C_in/RConn1 -- PV Array1/RConn2 -- Voltage Measurement/LConn2
  C_in/LConn1 -- L_boost/LConn1 -- PV Array1/RConn1
  RC_out/LConn1 -- Boost Converter/RConn1 -- Voltage Measurement/LConn1 -- Two-Level Converter/RConn1
  C/RConn1 -- Two-Level Converter/LConn3
  B/RConn1 -- Two-Level Converter/LConn2
  L_boost/RConn1 -- Boost Converter/LConn1

== system Integration_1_1/Subsystem14 ==
  Parallel RLC Branch : spsParallelRLCBranchLib/Parallel RLC Branch  LConnTagsString=a  RConnTagsString=__new0  BranchType=RC  Resistance=100  Inductance=1e-3  SetiL0=off  InitialCurrent=0  Capacitance=0.54e-6  Setx0=off  InitialVoltage=0  Measurements=None
  Parallel RLC Branch1 : spsParallelRLCBranchLib/Parallel RLC Branch  LConnTagsString=a  RConnTagsString=__new0  BranchType=RC  Resistance=100  Inductance=1e-3  SetiL0=off  InitialCurrent=0  Capacitance=0.54e-6  Setx0=off  InitialVoltage=0  Measurements=None
  Parallel RLC Branch2 : spsParallelRLCBranchLib/Parallel RLC Branch  LConnTagsString=a  RConnTagsString=__new0  BranchType=RC  Resistance=100  Inductance=1e-3  SetiL0=off  InitialCurrent=0  Capacitance=0.54e-6  Setx0=off  InitialVoltage=0  Measurements=None
  Three-Phase Series RLC Branch1 : spsThreePhaseSeriesRLCBranchLib/Three-Phase Series RLC Branch  LConnTagsString=A|B|C  RConnTagsString=A|B|C  BranchType=L  Resistance=1  Inductance=3*5.56e-3  Capacitance=1e-6  Measurements=None
  A : PMIOPort  Side=Left
  B : PMIOPort  Port=2  Side=Left
  C : PMIOPort  Port=3  Side=Left
  a : PMIOPort  Port=4  Side=Right
  b : PMIOPort  Port=5  Side=Right
  c : PMIOPort  Port=6  Side=Right
  connections:
  b/RConn1 -- Three-Phase Series RLC Branch1/RConn2 -- Parallel RLC Branch2/LConn1 -- Parallel RLC Branch/RConn1
  Three-Phase Series RLC Branch1/RConn3 -- c/RConn1 -- Parallel RLC Branch2/RConn1 -- Parallel RLC Branch1/LConn1
  a/RConn1 -- Three-Phase Series RLC Branch1/RConn1 -- Parallel RLC Branch/LConn1 -- Parallel RLC Branch1/RConn1
  Three-Phase Series RLC Branch1/LConn1 -- A/RConn1
  Three-Phase Series RLC Branch1/LConn2 -- B/RConn1
  Three-Phase Series RLC Branch1/LConn3 -- C/RConn1

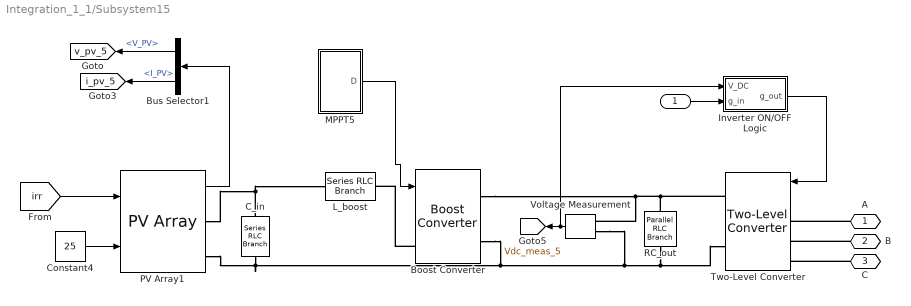
== system Integration_1_1/Subsystem15 ==
  "  " : Inport
  Boost Converter : spsBoostConverterLib/Boost Converter  ModelType=Average model (D-controlled)  Ron=1e-3  Rs=1e6  Cs=inf  Vforward=[0,0]  Ron_Diode=1e-3  Rs_Diode=1e6  Cs_Diode=inf  Vf_Diode=1e-3  Rs_CurrentSource=inf  Ron_ACsource=1e-3
      settings: LibrarySourceBlock=sps_lib/Power Electronics/Boost Converter
  Bus Selector1 : BusSelector  OutputSignals=V_PV,I_PV
  C_in : spsSeriesRLCBranchLib/Series RLC Branch  LConnTagsString=__new0  RConnTagsString=__new0  BranchType=C  Resistance=1e-5  Inductance=1e-3  SetiL0=off  InitialCurrent=0  Capacitance=418e-6  Setx0=off  InitialVoltage=426.5  Measurements=Branch voltage and current
  Constant4 : Constant  Value=25
  Inverter ON/OFF Logic : Subsystem
  L_boost : spsSeriesRLCBranchLib/Series RLC Branch  LConnTagsString=__new0  RConnTagsString=__new0  BranchType=L  Resistance=1e-3  Inductance=117.45e-3  SetiL0=off  InitialCurrent=0  Capacitance=100e-6  Setx0=off  InitialVoltage=230  Measurements=None
  MPPT5 : Subsystem
  PV Array1 : spsPVArrayLib/PV Array  Npar=4  Nser=5  PlotType=array @ 1000 W/m2 & specified temperatures  S_vec="[ 1000  500  100 ]"  Temp_C_vec="[ 45 25  ]"  ModuleName=SunPower SPR-415E-WHT-D  PlotWhenSelected=off  Pm=414.801  Ncell=128  Voc=85.3  Isc=6.09  Vm=72.9  Im=5.69  beta_Voc_pc=-0.229  alpha_Isc_pc=0.030706  beta_Voc=-0.19534  alpha_Isc=0.00187  IL=6.0978  I0=7.1698e-13  nI=0.87223  Rsh=419.7781  Rs=0.53711  RobustModel=off  RobustCellTemperature=313.3991  BAL=on  Tc=1e-6  Tfilter=5e-5
  RC_out : spsParallelRLCBranchLib/Parallel RLC Branch  LConnTagsString=a  RConnTagsString=__new0  BranchType=RC  Resistance=50  Inductance=1e-3  SetiL0=off  InitialCurrent=0  Capacitance=318.7e-6  Setx0=off  InitialVoltage=700  Measurements=None
  Two-Level Converter : spsTwoLevelConverterLib/Two-Level Converter  ModelType=Average model (No rectifier mode)  Ron=1e-3  Rs=1e6  Cs=inf  Vforward=[0,0]  Ron_Diode=1e-3  Rs_Diode=1e6  Cs_Diode=inf  Vf_Diode=1e-3  Rs_CurrentSource=inf  Ron_ACsource=1e-3
  Voltage Measurement : spsVoltageMeasurementLib/Voltage Measurement  PhasorSimulation=off  OutputType=Complex  PSBequivalent=0
  A : PMIOPort  Side=Left
  B : PMIOPort  Port=2  Side=Left
  C : PMIOPort  Port=3  Side=Left
  tag scope: Vdc_meas_5=global, i_pv_5=global, v_pv_5=global
  wires:
  Bus Selector1/1 -> [v_pv_5]  "<V_PV>"
  Constant4/1 -> PV Array1/2
  Bus Selector1/2 -> [i_pv_5]  "<I_PV>"
  PV Array1/1 -> Bus Selector1/1
  [irr] -> PV Array1/1
  Voltage Measurement/1 -> Inverter ON/OFF Logic/1(V_DC), [Vdc_meas_5]
  Inverter ON/OFF Logic/1(g_out) -> Two-Level Converter/1
  "  "/1 -> Inverter ON/OFF Logic/2(g_in)
  MPPT5/1(D) -> Boost Converter/1
  connections:
  A/RConn1 -- Two-Level Converter/LConn1
  Two-Level Converter/RConn2 -- RC_out/RConn1 -- Voltage Measurement/LConn2 -- Boost Converter/RConn2 -- C_in/RConn1 -- PV Array1/RConn2
  C_in/LConn1 -- L_boost/LConn1 -- PV Array1/RConn1
  RC_out/LConn1 -- Boost Converter/RConn1 -- Voltage Measurement/LConn1 -- Two-Level Converter/RConn1
  C/RConn1 -- Two-Level Converter/LConn3
  B/RConn1 -- Two-Level Converter/LConn2
  Boost Converter/LConn1 -- L_boost/RConn1

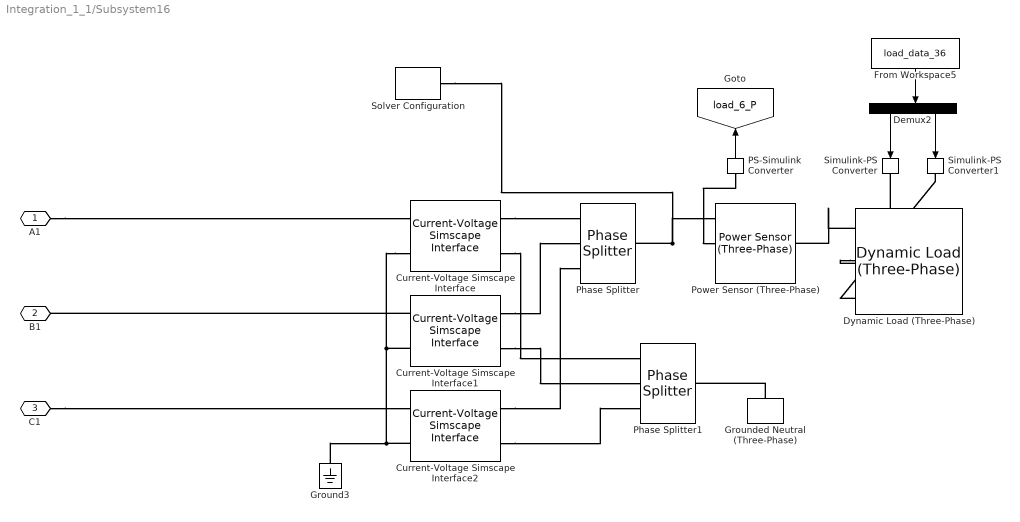
== system Integration_1_1/Subsystem16 ==
  Current-Voltage Simscape Interface : spsCurrentVoltageSimscapeInterfaceLib/Current-Voltage Simscape Interface  DFT=off  FMode=Low pass filter (continuous)  T=1e-4  Ts=50e-6  i0=0  v0=0  Sd=Specialized Power Systems side  Measurements=off
  Current-Voltage Simscape Interface1 : spsCurrentVoltageSimscapeInterfaceLib/Current-Voltage Simscape Interface  DFT=off  FMode=Low pass filter (continuous)  T=1e-4  Ts=50e-6  i0=0  v0=0  Sd=Specialized Power Systems side  Measurements=off
  Current-Voltage Simscape Interface2 : spsCurrentVoltageSimscapeInterfaceLib/Current-Voltage Simscape Interface  DFT=off  FMode=Low pass filter (continuous)  T=1e-4  Ts=50e-6  i0=0  v0=0  Sd=Specialized Power Systems side  Measurements=off
  Demux2 : Demux  Outputs=2
  Dynamic Load (Three-Phase) : ee_lib/Passive/Dynamic Load (Three-Phase)  port_option=ee.enum.threePhasePort.composite  FRated=50 Hz  Vline_rms_min=400 V  tau=0.01 s  Vline_rms_ini=400 V  Vang_ini=0 deg  gmin=0 S  fault_action=simscape.enum.assert.action.none  t_fault=1 s
      settings: InternalSimscapePortConfiguration="{\"Bottom\":[],\"Left\":[{\"id\":\"N\",\"label\":\"~\",\"type\":\"foundation.electrical.three_phase\"}],\"Right\":[],\"Top\":[{\"id\":\"P\",\"label\":\"P\",\"type\":\"input\"},{\"id\":\"Q\",\"label\":\"Q\",\"type\":\"input\"}]}"
  From Workspace5 : FromWorkspace  VariableName=load_data_36  SampleTime=0.01
  Ground3 : spsGroundLib/Ground  LConnTagsString=a
  Grounded Neutral (Three-Phase) : ee_lib/Connectors & References/Grounded Neutral (Three-Phase)
  PS-Simulink Converter : nesl_utility/PS-Simulink Converter  PhysicalDomain=network_engine_domain  SubClassName=ps_output  LeftPortType=input  RightPortType=output  PseudoPeriodic=off  Frequencies=[]  VectorFormat=inherit  Unit=inherit  AffineConversion=off
  Phase Splitter : ee_lib/Connectors & References/Phase Splitter
  Phase Splitter1 : ee_lib/Connectors & References/Phase Splitter
  Power Sensor (Three-Phase) : ee_lib/Sensors & Transducers/Power Sensor (Three-Phase)  load_type=ee.enum.passive.type_balanced.unbalanced  f0=50 Hz  config=ee.enum.with_neutral.no  rho=1
      settings: InternalSimscapePortConfiguration="{\"Bottom\":[],\"Left\":[{\"id\":\"N1\",\"label\":\"~1\",\"type\":\"foundation.electrical.three_phase\"}],\"Right\":[{\"id\":\"N2\",\"label\":\"~2\",\"type\":\"foundation.electrical.three_phase\"}],\"Top\":[{\"id\":\"Pm\",\"label\":\"P\",\"type\":\"output\"},{\"id\":\"Qm\",\"label\":\"Q\",\"type\":\"output\"}]}"
  Simulink-PS Converter : nesl_utility/Simulink-PS Converter  PhysicalDomain=network_engine_domain  SubClassName=ps_input  LeftPortType=input  RightPortType=output  PseudoPeriodic=off  Frequencies=[]  NoiseDistribution=none  NoiseParameters=[]  Unit=1  AffineConversion=off  FilteringAndDerivatives=provide  SimscapeFilterOrder=1  InputFilterTimeConstant=0.001  UdotUserProvided=0
  Simulink-PS Converter1 : nesl_utility/Simulink-PS Converter  PhysicalDomain=network_engine_domain  SubClassName=ps_input  LeftPortType=input  RightPortType=output  PseudoPeriodic=off  Frequencies=[]  NoiseDistribution=none  NoiseParameters=[]  Unit=1  AffineConversion=off  FilteringAndDerivatives=provide  SimscapeFilterOrder=1  InputFilterTimeConstant=0.001  UdotUserProvided=0
  Solver Configuration : nesl_utility/Solver Configuration  PhysicalDomain=network_engine_domain  SubClassName=solver  LeftPortType=input  RightPortType=generic  Tones=[]  Harmonics=[]  SimulateNoise=off  Profile=off  UseLocalSampling=off  EnableSwitchedLinearOptims=on  FrequencyDomain=off  UseCCode=off  RelTol=0.001  AbsTol=0.001  MinStep=1e-09  ToWorkspace=off  RevertToSquareIcSolve=off  NumHomotopyIterations=100  PhasorMode=off  PhasorModeNumHarmonics=1  ConsistencySolver=NEWTON_XTOL_AFTER_FTOL  IndexReductionMethod=DerivativeReplacement  DoDC=on  ResidualTolerance=1e-09  ConsistencyTolSource=GLOBAL  ConsistencyAbsTol=0.001  ConsistencyRelTol=0.001  ConsistencyTolFactor=0.001  UseLocalSolver=off  LocalSolverChoice=NE_BACKWARD_EULER_ADVANCER  ResolveIndetEquations=on  FunctionEvalNumThread=1  LocalSolverSampleTime=0.0001  DoFixedCost=off  MaxNonlinIter=3  MaxModeIter=2  ComputeImpulses=off  ImpulseIterations=2  LinearAlgebra=Sparse  LinearAlgebraNumThread=0  EquationFormulation=NE_TIME_EF  DelaysMemoryBudget=1024  AutomaticFiltering=off  FilteringTimeConstant=0.001  PartitionStorageMethod=AS_NEEDED  PartitionMemoryBudget=1024  PartitionMethod=ROBUST  MultibodyUseLocalSolver=off  MultibodyLocalSolverChoice=ODE1  MultibodyLocalSolverSampleTime=0.001
  A1 : PMIOPort  Side=Left
  B1 : PMIOPort  Port=2  Side=Left
  C1 : PMIOPort  Port=3  Side=Left
  tag scope: load_6_P=global
  wires:
  Demux2/1 -> Simulink-PS Converter/1
  PS-Simulink Converter/1 -> [load_6_P]
  Demux2/2 -> Simulink-PS Converter1/1
  From Workspace5/1 -> Demux2/1
  connections:
  C1/RConn1 -- Current-Voltage Simscape Interface2/LConn1
  Current-Voltage Simscape Interface/LConn2 -- Ground3/LConn1 -- Current-Voltage Simscape Interface2/LConn2 -- Current-Voltage Simscape Interface1/LConn2
  Current-Voltage Simscape Interface1/LConn1 -- B1/RConn1
  A1/RConn1 -- Current-Voltage Simscape Interface/LConn1
  Dynamic Load (Three-Phase)/LConn2 -- Simulink-PS Converter/RConn1
  PS-Simulink Converter/LConn1 -- Power Sensor (Three-Phase)/LConn2
  Current-Voltage Simscape Interface/RConn2 -- Phase Splitter1/RConn1
  Grounded Neutral (Three-Phase)/LConn1 -- Phase Splitter1/LConn1
  Dynamic Load (Three-Phase)/LConn3 -- Simulink-PS Converter1/RConn1
  Current-Voltage Simscape Interface/RConn1 -- Phase Splitter/RConn1
  Current-Voltage Simscape Interface2/RConn1 -- Phase Splitter/RConn3
  Current-Voltage Simscape Interface1/RConn1 -- Phase Splitter/RConn2
  Dynamic Load (Three-Phase)/LConn1 -- Power Sensor (Three-Phase)/RConn1
  Current-Voltage Simscape Interface2/RConn2 -- Phase Splitter1/RConn3
  Current-Voltage Simscape Interface1/RConn2 -- Phase Splitter1/RConn2
  Phase Splitter/LConn1 -- Solver Configuration/RConn1 -- Power Sensor (Three-Phase)/LConn1

== system Integration_1_1/Subsystem17 ==
  Parallel RLC Branch : spsParallelRLCBranchLib/Parallel RLC Branch  LConnTagsString=a  RConnTagsString=__new0  BranchType=RC  Resistance=85  Inductance=1e-3  SetiL0=off  InitialCurrent=0  Capacitance=0.655e-6  Setx0=off  InitialVoltage=0  Measurements=None
  Parallel RLC Branch1 : spsParallelRLCBranchLib/Parallel RLC Branch  LConnTagsString=a  RConnTagsString=__new0  BranchType=RC  Resistance=85  Inductance=1e-3  SetiL0=off  InitialCurrent=0  Capacitance=0.655e-6  Setx0=off  InitialVoltage=0  Measurements=None
  Parallel RLC Branch2 : spsParallelRLCBranchLib/Parallel RLC Branch  LConnTagsString=a  RConnTagsString=__new0  BranchType=RC  Resistance=85  Inductance=1e-3  SetiL0=off  InitialCurrent=0  Capacitance=0.655e-6  Setx0=off  InitialVoltage=0  Measurements=None
  Three-Phase Series RLC Branch1 : spsThreePhaseSeriesRLCBranchLib/Three-Phase Series RLC Branch  LConnTagsString=A|B|C  RConnTagsString=A|B|C  BranchType=L  Resistance=1  Inductance=3*4.63e-3  Capacitance=1e-6  Measurements=None
  A : PMIOPort  Side=Left
  B : PMIOPort  Port=2  Side=Left
  C : PMIOPort  Port=3  Side=Left
  a : PMIOPort  Port=4  Side=Right
  b : PMIOPort  Port=5  Side=Right
  c : PMIOPort  Port=6  Side=Right
  connections:
  c/RConn1 -- Three-Phase Series RLC Branch1/RConn3 -- Parallel RLC Branch2/LConn1 -- Parallel RLC Branch1/RConn1
  Three-Phase Series RLC Branch1/LConn3 -- C/RConn1
  Three-Phase Series RLC Branch1/LConn2 -- B/RConn1
  Three-Phase Series RLC Branch1/LConn1 -- A/RConn1
  a/RConn1 -- Parallel RLC Branch2/RConn1 -- Parallel RLC Branch/LConn1 -- Three-Phase Series RLC Branch1/RConn1
  b/RConn1 -- Parallel RLC Branch1/LConn1 -- Parallel RLC Branch/RConn1 -- Three-Phase Series RLC Branch1/RConn2

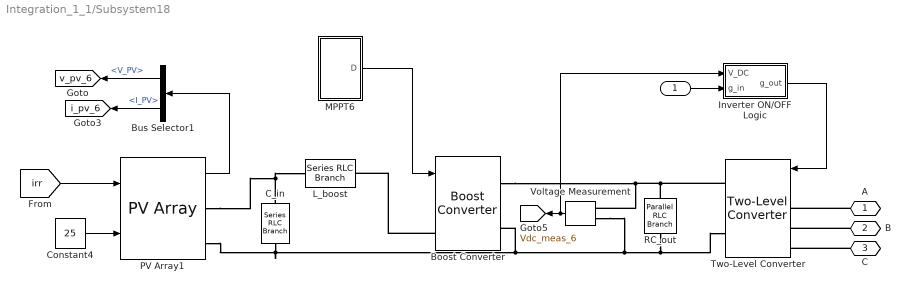
== system Integration_1_1/Subsystem18 ==
  "  " : Inport
  Boost Converter : spsBoostConverterLib/Boost Converter  ModelType=Average model (D-controlled)  Ron=1e-3  Rs=1e6  Cs=inf  Vforward=[0,0]  Ron_Diode=1e-3  Rs_Diode=1e6  Cs_Diode=inf  Vf_Diode=1e-3  Rs_CurrentSource=inf  Ron_ACsource=1e-3
      settings: LibrarySourceBlock=sps_lib/Power Electronics/Boost Converter
  Bus Selector1 : BusSelector  OutputSignals=V_PV,I_PV
  C_in : spsSeriesRLCBranchLib/Series RLC Branch  LConnTagsString=__new0  RConnTagsString=__new0  BranchType=C  Resistance=1e-5  Inductance=1e-3  SetiL0=off  InitialCurrent=0  Capacitance=241.03e-6  Setx0=off  InitialVoltage=426.5  Measurements=Branch voltage and current
  Constant4 : Constant  Value=25
  Inverter ON/OFF Logic : Subsystem
  L_boost : spsSeriesRLCBranchLib/Series RLC Branch  LConnTagsString=__new0  RConnTagsString=__new0  BranchType=L  Resistance=1e-3  Inductance=100e-3  SetiL0=off  InitialCurrent=0  Capacitance=100e-6  Setx0=off  InitialVoltage=230  Measurements=None
  MPPT6 : Subsystem
  PV Array1 : spsPVArrayLib/PV Array  Npar=4  Nser=6  PlotType=array @ 1000 W/m2 & specified temperatures  S_vec="[ 1000  500  100 ]"  Temp_C_vec="[ 45 25  ]"  ModuleName=SunPower SPR-415E-WHT-D  PlotWhenSelected=off  Pm=414.801  Ncell=128  Voc=85.3  Isc=6.09  Vm=72.9  Im=5.69  beta_Voc_pc=-0.229  alpha_Isc_pc=0.030706  beta_Voc=-0.19534  alpha_Isc=0.00187  IL=6.0978  I0=7.1698e-13  nI=0.87223  Rsh=419.7781  Rs=0.53711  RobustModel=off  RobustCellTemperature=313.3991  BAL=on  Tc=1e-6  Tfilter=5e-5
  RC_out : spsParallelRLCBranchLib/Parallel RLC Branch  LConnTagsString=a  RConnTagsString=__new0  BranchType=C  Resistance=5  Inductance=1e-3  SetiL0=off  InitialCurrent=0  Capacitance=220e-6  Setx0=off  InitialVoltage=700  Measurements=None
  Two-Level Converter : spsTwoLevelConverterLib/Two-Level Converter  ModelType=Average model (No rectifier mode)  Ron=1e-3  Rs=1e6  Cs=inf  Vforward=[0,0]  Ron_Diode=1e-3  Rs_Diode=1e6  Cs_Diode=inf  Vf_Diode=1e-3  Rs_CurrentSource=inf  Ron_ACsource=1e-3
  Voltage Measurement : spsVoltageMeasurementLib/Voltage Measurement  PhasorSimulation=off  OutputType=Complex  PSBequivalent=0
  A : PMIOPort  Side=Left
  B : PMIOPort  Port=2  Side=Left
  C : PMIOPort  Port=3  Side=Left
  tag scope: Vdc_meas_6=global, i_pv_6=global, v_pv_6=global
  wires:
  Bus Selector1/1 -> [v_pv_6]  "<V_PV>"
  Constant4/1 -> PV Array1/2
  Bus Selector1/2 -> [i_pv_6]  "<I_PV>"
  PV Array1/1 -> Bus Selector1/1
  [irr] -> PV Array1/1
  Inverter ON/OFF Logic/1(g_out) -> Two-Level Converter/1
  MPPT6/1(D) -> Boost Converter/1
  Voltage Measurement/1 -> Inverter ON/OFF Logic/1(V_DC), [Vdc_meas_6]
  "  "/1 -> Inverter ON/OFF Logic/2(g_in)
  connections:
  A/RConn1 -- Two-Level Converter/LConn1
  Two-Level Converter/RConn2 -- RC_out/RConn1 -- Voltage Measurement/LConn2 -- C_in/RConn1 -- PV Array1/RConn2 -- Boost Converter/RConn2
  C_in/LConn1 -- L_boost/LConn1 -- PV Array1/RConn1
  RC_out/LConn1 -- Boost Converter/RConn1 -- Voltage Measurement/LConn1 -- Two-Level Converter/RConn1
  C/RConn1 -- Two-Level Converter/LConn3
  B/RConn1 -- Two-Level Converter/LConn2
  Boost Converter/LConn1 -- L_boost/RConn1

== system Integration_1_1/Subsystem2 ==
  "  " : Inport
  Boost Converter : spsBoostConverterLib/Boost Converter  ModelType=Average model (D-controlled)  Ron=1e-3  Rs=1e6  Cs=inf  Vforward=[0,0]  Ron_Diode=1e-3  Rs_Diode=1e6  Cs_Diode=inf  Vf_Diode=1e-3  Rs_CurrentSource=inf  Ron_ACsource=1e-3
  Bus Selector1 : BusSelector  OutputSignals=V_PV,I_PV
  C_in : spsSeriesRLCBranchLib/Series RLC Branch  LConnTagsString=__new0  RConnTagsString=__new0  BranchType=C  Resistance=1e-5  Inductance=1e-3  SetiL0=off  InitialCurrent=0  Capacitance=525e-6  Setx0=off  InitialVoltage=426.5  Measurements=Branch voltage and current
  Constant4 : Constant  Value=25
  Inverter ON/OFF Logic : Subsystem
  L_boost : spsSeriesRLCBranchLib/Series RLC Branch  LConnTagsString=__new0  RConnTagsString=__new0  BranchType=L  Resistance=1e-3  Inductance=95e-3  SetiL0=off  InitialCurrent=0  Capacitance=100e-6  Setx0=off  InitialVoltage=230  Measurements=None
  MPPT2 : Subsystem
  PV Array1 : spsPVArrayLib/PV Array  Npar=5  Nser=5  PlotType=array @ 1000 W/m2 & specified temperatures  S_vec="[ 1000  500  100 ]"  Temp_C_vec="[ 45 25  ]"  ModuleName=SunPower SPR-415E-WHT-D  PlotWhenSelected=off  Pm=414.801  Ncell=128  Voc=85.3  Isc=6.09  Vm=72.9  Im=5.69  beta_Voc_pc=-0.229  alpha_Isc_pc=0.030706  beta_Voc=-0.19534  alpha_Isc=0.00187  IL=6.0978  I0=7.1698e-13  nI=0.87223  Rsh=419.7781  Rs=0.53711  RobustModel=off  RobustCellTemperature=313.3991  BAL=on  Tc=1e-6  Tfilter=5e-5
  RC_out : spsParallelRLCBranchLib/Parallel RLC Branch  LConnTagsString=a  RConnTagsString=__new0  BranchType=C  Resistance=10  Inductance=1e-3  SetiL0=off  InitialCurrent=0  Capacitance=6*398e-6  Setx0=off  InitialVoltage=700  Measurements=None
  Two-Level Converter : spsTwoLevelConverterLib/Two-Level Converter  ModelType=Average model (No rectifier mode)  Ron=1e-3  Rs=1e6  Cs=inf  Vforward=[0,0]  Ron_Diode=1e-3  Rs_Diode=1e6  Cs_Diode=inf  Vf_Diode=1e-3  Rs_CurrentSource=inf  Ron_ACsource=1e-3
  Voltage Measurement : spsVoltageMeasurementLib/Voltage Measurement  PhasorSimulation=off  OutputType=Complex  PSBequivalent=0
  A : PMIOPort  Side=Left
  B : PMIOPort  Port=2  Side=Left
  C : PMIOPort  Port=3  Side=Left
  tag scope: Vdc_meas_2=global, i_pv_2=global, v_pv_2=global
  wires:
  Voltage Measurement/1 -> [Vdc_meas_2], Inverter ON/OFF Logic/1(V_DC)
  "  "/1 -> Inverter ON/OFF Logic/2(g_in)
  Inverter ON/OFF Logic/1(g_out) -> Two-Level Converter/1
  MPPT2/1(D) -> Boost Converter/1
  [irr] -> PV Array1/1
  PV Array1/1 -> Bus Selector1/1
  Bus Selector1/2 -> [i_pv_2]  "<I_PV>"
  Constant4/1 -> PV Array1/2
  Bus Selector1/1 -> [v_pv_2]  "<V_PV>"
  connections:
  L_boost/RConn1 -- Boost Converter/LConn1
  B/RConn1 -- Two-Level Converter/LConn2
  C/RConn1 -- Two-Level Converter/LConn3
  Voltage Measurement/LConn1 -- Boost Converter/RConn1 -- Two-Level Converter/RConn1 -- RC_out/LConn1
  PV Array1/RConn1 -- L_boost/LConn1 -- C_in/LConn1
  PV Array1/RConn2 -- C_in/RConn1 -- Boost Converter/RConn2 -- Voltage Measurement/LConn2 -- RC_out/RConn1 -- Two-Level Converter/RConn2
  A/RConn1 -- Two-Level Converter/LConn1
